simulink model "RobotX_ss_acousticsSKIP_dock_odoa_1021"  (R2014a)
settings: Solver=FixedStepDiscrete  StartTime=0.0  StopTime=inf  FixedStep=.25  RelTol=1e-3
undefined symbols (not defined in the file): Com1, Com2, Com3, Com4, DiscIntNeverNeededParam, standard
libraries: xpcseriallib x42, slrtlib x8, simulink x7, speedgoatlib x2, speedgoatlib_IO102 x1
(part 7 of 19)

== matlab function RobotX_ss_acousticsSKIP_dock_odoa_1021/Main FSM/ODOA/SLAM1/SLAM enabled/slammed ==
  data: mpa output; lm_data input; pre_part_positions input; part_positions output; positionboat input
%% SLAM by Chidananda Matada Shivananda
%  Copyright 2010 Randolph Voorhies

%  Edited 2014 Nick DiLeo - Modifications for unknown data association
%  and multiple measurements in a single timestep
    
%  Edited 2014 Chidananda Matada Shivananda - Simulink compatability, New
%  clustering technique added

%  This program is free software: you can redistribute it and/or modify
%  it under the terms of the GNU General Public License as published by
%  the Free Software Foundation, either version 3 of the License, or
%  (at your option) any later version.
%
%  This program is distributed in the hope that it will be useful,
%  but WITHOUT ANY WARRANTY; without even the implied warranty of
%  MERCHANTABILITY or FITNESS FOR A PARTICULAR PURPOSE.  See the
%  GNU General Public License for more details.
%
%  You should have received a copy of the GNU General Public License
%  along with this program.  If not, see <http://www.gnu.org/licenses/>.

function [mpa,part_positions]   = slammed(lm_data,pre_part_positions,positionboat)

%% General comments

% the angles in radians
% the ditance in m

%% Initialisations.

persistent particles avg_robot;
num_particles = 50;

% the limits
max_read_distance = 10;
min_read_distance = 5;
min_read_angle = -67.5*pi/180; %radians- maximum read angle
max_read_angle = 67.5*pi/180;

% The initial starting position of the robot Use UTM coordinates from GPS
avg_robot_position = [0;0;0];% x y rotation

% The Gaussian variance of the movement commands
% Approximating there are only two drives
% movement_variance = [.1;.1];   % Left drive Right_drive
% M = [movement_variance(1), 0.0;
%      0.0, movement_variance(2)];
measurement_variance = [0.01; 0.01];   % Distance Angle
R = [measurement_variance(1), 0.0;
    0.0, measurement_variance(2)];

default_importance=0.001;

if isempty(particles)
    %  Particles
    %             w[1]
    %             position[1,3]
    %             num_landmarks[300] this is to keep history
    
    %             lm_weight[2,15]based on number of landmarks
    %             landmarks[15]
    %                         position[2,1]
    %                         E[2,2]
    %                         counter[1]
    particles=repmat(struct('w',1.0/num_particles,'position',avg_robot_position,'num_landmarks',zeros(1,2),'lm_weight',repmat(1.0/num_particles,10,15),'landmarks',repmat(struct('pos',zeros(1,2),'E',zeros(2,2),'counter',0),1,15)),1,50);
    avg_robot_position = average_pos(particles,num_particles);
end

if isempty(avg_robot)
    avg_robot=avg_robot_position;
end

avg_robot_position=avg_robot;

%% Upload the moved data onto the particles
for shiva9=1:50
    particles(shiva9).position(1)= pre_part_positions(3*(shiva9-1)+1);
    particles(shiva9).position(2)= pre_part_positions(3*(shiva9-1)+1)*(pi/180);
    particles(shiva9).position(3)= pre_part_positions(3*(shiva9-1)+1);
end

%% Try to take a reading from each landmark and calculate the Jacobian
doResample = false;
% The input got from landmarks
[~,cols]=find(lm_data ~= 0);
if (isempty(cols)==0)% if the cols is not empty
    doResample=true; %if there is new measurement, then resample particles
end

if (doResample==true)
%     [r,~]=size(cols);
    [~,r]=size(cols);
    shiva=1;
    G=zeros(2,2,ceil(r/2));
    z_real=zeros(2,ceil(r/2));
    read_distance=zeros(ceil(r/2));
    read_angle=zeros(ceil(r/2));
    
    for lIdx = 1:2:r %amount of visible landmarks
        real_landmark = [lm_data(cols(lIdx+1)),lm_data(cols(lIdx))];
        % Take a real (noisy) measurement from the robot to the landmark
        %         [z_real(:,lIdx), G(:,:,lIdx)] = getRealMeasurement(avg_robot_position, real_landmark, [0 0]);
        %         function [z, H] = getRealMeasurement(pos, landmark_pos, observation_variance)
        
        landmark_angle=real_landmark(1);
        landmark_distance=real_landmark(2);
        % Compute the Jacobian of this measurement function
        q = landmark_distance^2.0;
        G(:,:,shiva) = [-(real_landmark(1) - avg_robot_position(1))/sqrt(q), -(real_landmark(2) - avg_robot_position(2))/sqrt(q);
            (real_landmark(2) - avg_robot_position(2))/q,       -(real_landmark(1) - avg_robot_position(1))/q];
        
        z_real(:,shiva) = [landmark_distance; landmark_angle];
        read_distance(shiva) = z_real(1,shiva);
        read_angle(shiva)    = z_real(2,shiva);
        shiva=shiva+1;
    end
    %     shiva=1;
    
    for pIdx = 1:num_particles
        %     particles(pIdx).lm_weight=[];
        %     clear z_p H Q
        %         coder.varsize('H', [2,2,16],[0 0 1]);
        num_landmarks=particles(pIdx).num_landmarks(1);
        assert(num_landmarks<20);
        H=zeros(2,2,num_landmarks);
        %         coder.varsize('z_p', [2 1 16]);
        z_p=zeros(2,1,num_landmarks);
        Q=zeros(2,2,num_landmarks);
        for j=1:particles(pIdx).num_landmarks(1)
            %             [z_p(:,j), H(:,:,j)] = getMeasurement(particles(pIdx).position, particles(pIdx).landmarks(j).pos, [0 0]);
            %             function [z, H] = getRealMeasurement(pos, landmark_pos, observation_variance)
            landmark_angle=particles(pIdx).landmarks(j).pos(1);
            landmark_distance=particles(pIdx).landmarks(j).pos(2);
            
            % Compute the Jacobian of this measurement function
            q = landmark_distance^2.0;
            %   H = [-(landmark_pos(1) - pos(1))/sqrt(q), -(landmark_pos(2) - pos(2))/sqrt(q), 0.0;
            %         (landmark_pos(2) - pos(2))/q,       -(landmark_pos(1) - pos(1))/q,      -1.0;
            %         0.0,                                0.0,                               1.0];
            
            H(:,:,j) = [-(particles(pIdx).landmarks(j).pos(1) - particles(pIdx).position(1))/sqrt(q), -(particles(pIdx).landmarks(j).pos(2) - particles(pIdx).position(2))/sqrt(q);
                (particles(pIdx).landmarks(j).pos(2) - particles(pIdx).position(2))/q,       -(particles(pIdx).landmarks(j).pos(1) - particles(pIdx).position(1))/q];
            
            
            z_p(:,j) = [landmark_distance;
                landmark_angle];
            
            for measured_lm=1:size(z_real,2)
                residual = z_real(:,measured_lm) - z_p(:,j);
                Q(:,:,j) = H(:,:,j)' * particles(pIdx).landmarks(j).E * H(:,:,j) + R;
                particles(pIdx).lm_weight(measured_lm,j) = particles(pIdx).w * norm(2*pi*Q(:,:,j)).^(-1/2)*exp(-1/2*(residual'/Q(:,:,j)*residual));
            end
        end
        
        particles(pIdx).num_landmarks(2)=particles(pIdx).num_landmarks(1);
        num_landmarks2=particles(pIdx).num_landmarks(2);
        assert(num_landmarks2<20);
        
        %           clear c_hat
        %         clear cost_table data_associate_mat data_associate_vect
        %%%%%%%%%%%%%%%%%%%%%%%%%%%%%%%%%%%%%%%%%%%%%%%%%%%%%%%%%%%%%%%%%%%%%%%%%%%%%%%%%%%%%%%%%%%%%%%%%%%%%%%%%%%%%%%%%%%%%%%%%%%%%%%%%%%%%%%%%%%%%
        cost_table=zeros(size(z_real,2),num_landmarks+size(z_real,2));
        %         cost_table=zeros(size(z_real,2),num_landmarks);
        
        if (num_landmarks~=0)
            cost_table(1:size(z_real,2),1:particles(pIdx).num_landmarks(1))=particles(pIdx).lm_weight(1:size(z_real,2),1:particles(pIdx).num_landmarks(1));
        end
        cost_table(1:size(z_real,2),particles(pIdx).num_landmarks(1)+1:particles(pIdx).num_landmarks(1)+size(z_real,2)) =default_importance*eye(size(z_real,2));
        
        particles(pIdx).w=max(max(cost_table,[],1),[],2);
        [~, idx_hold]=max(cost_table,[],1); %this is the max correseponding for each measurement
        for i=1:size(cost_table,2)
            idx_zero=setdiff(1:size(cost_table,1),idx_hold(i));
            cost_table(idx_zero,i)=0;
        end
        
        cost_table1=cost_table;
        for shiva14=1:size(cost_table,2)
            cost_table(:,shiva14)=cost_table1(:,size(cost_table,2)-shiva14+1);
        end
        
        
        new_landmarks=0;
        for measured_lm=1:size(z_real,2)
            [~, IDX] = max(cost_table(measured_lm,:));
            if IDX > particles(pIdx).num_landmarks(1)
                new_landmarks=new_landmarks+1;
            end
        end
        
        
        assert(new_landmarks<20);
        data_associate_mat=zeros(size(z_real,2),new_landmarks+num_landmarks2);
        
        for measured_lm=1:size(z_real,2)
            [~, IDX] = max(cost_table(measured_lm,:));
            if IDX > particles(pIdx).num_landmarks(1)
                %we haven't seen this landmark before
                %                 if particles(pIdx).num_landmarks(2)>14
                %                     break;
                %                 end
                particles(pIdx).num_landmarks(2)=particles(pIdx).num_landmarks(2)+1; %add new landmark
                data_associate_mat(measured_lm,particles(pIdx).num_landmarks(2))=measured_lm; %set correspondance b/t measurement and feature j
            else
                %we've already seen this landmark
                %           [val idx]=max(particles(pIdx).lm_weight(measured_lm,:));
                data_associate_mat(measured_lm,IDX)=measured_lm; %measurement is a known feature
            end
            
        end
        
        num_landmarks2=particles(pIdx).num_landmarks(2);
        assert(num_landmarks2<20);
        Hn=zeros(2,2,num_landmarks2);
        t=size(H);
        for i=1:t(3)
            Hn(:,:,i)=H(:,:,i);
        end
        
        %         H=zeros(2,2,num_landmarks2);
        H=Hn;
        
        data_associate_vect=max(data_associate_mat,[],1); %vector that contains measurement correspondance to landmarks
        i=1;
        feature_to_delete=zeros(num_landmarks2);
        for j=1:particles(pIdx).num_landmarks(2) %length(data_associate_vect)
            if (data_associate_vect(j)>0 && j>particles(pIdx).num_landmarks(1))
                % If we have never seen this landmark, then we need to initialize it.
                % We'll just use whatever first reading we recieved.
                particles(pIdx).landmarks(j).pos = [particles(pIdx).position(1) + ...
                    sin(read_angle(data_associate_vect(j))+particles(pIdx).position(3))*read_distance(data_associate_vect(j));...
                    particles(pIdx).position(2) + cos(read_angle(data_associate_vect(j))+particles(pIdx).position(3))*read_distance(data_associate_vect(j))]';
                % Initialize the landmark position covariance
                H(:,:,j)=G(:,:,data_associate_vect(j));
                particles(pIdx).landmarks(j).E = inv(G(:,:,data_associate_vect(j)))' * R * inv(G(:,:,data_associate_vect(j)));
                particles(pIdx).landmarks(j).counter=1; %initialize counter
            elseif (data_associate_vect(j)>0 && j<=particles(pIdx).num_landmarks(1))
                %we've seen this landmark before
                K = particles(pIdx).landmarks(j).E * H(:,:,j) / Q(:,:,j);
                % Mix the ideal reading, and our actual reading using the Kalman gain, and use the result
                % to predict a new landmark position
                particles(pIdx).landmarks(j).pos = particles(pIdx).landmarks(j).pos + (K*(z_real(:,data_associate_vect(j))-z_p(:,j)))';
                % Update the covariance of this landmark
                particles(pIdx).landmarks(j).E = (eye(size(H(:,:,j))) - K*H(:,:,j)')*particles(pIdx).landmarks(j).E;
                particles(pIdx).landmarks(j).counter=particles(pIdx).landmarks(j).counter+1; %increment counter
            else
                % We are leaving these unchanged.  These are commented
                % out, but this is what is actually happening in alg.
                % particles(pIdx).landmarks(j).pos = particles(pIdx).landmarks(j).pos;
                % particles(pIdx).landmarks(j).E=particles(pIdx).landmarks(j).E;
                dist_to_landmark=norm([particles(pIdx).landmarks(j).pos(1)-particles(pIdx).position(1) particles(pIdx).landmarks(j).pos(2)-particles(pIdx).position(2)]);
                ang_to_landmark=atan2((particles(pIdx).landmarks(j).pos(1) - particles(pIdx).position(1)),...
                    (particles(pIdx).landmarks(j).pos(2) - particles(pIdx).position(2)))-particles(pIdx).position(3);
                if (dist_to_landmark > max_read_distance ||dist_to_landmark < min_read_distance || ang_to_landmark > max_read_angle || ang_to_landmark < min_read_angle)
                    %counter(pIdx,j)=counter(pIdx,j) %don't change counter
                else
                    particles(pIdx).landmarks(j).counter=particles(pIdx).landmarks(j).counter-1; %decrement counter
                    if particles(pIdx).landmarks(j).counter<0
                        feature_to_delete(i)=j; %we're going to delete all these features at the end of the loop
                        i=i+1;
                    end
                end
                %
            end %if
        end %end j
        %     'pos',zeros(1,2),'E',zeros(2,2),'counter',0
        if~(isempty(nonzeros(feature_to_delete)))
            tobe_del=nonzeros(feature_to_delete);
            for shiva4=1:length(feature_to_delete)
                particles(pIdx).landmarks(tobe_del(shiva4)).pos=zeros(1,2);
                particles(pIdx).landmarks(tobe_del(shiva4)).E=zeros(2,2);
                particles(pIdx).landmarks(tobe_del(shiva4)).counter=0;
            end
            particles(pIdx).num_landmarks(2)= particles(pIdx).num_landmarks(2)-length(tobe_del);
        end
        
        particles(pIdx).num_landmarks(1)=particles(pIdx).num_landmarks(2);
        
    end %pIdx
    
    particles=resample(particles) ;
    
    
    
end% if (doResample==true)


%% Clustering
landmarks_positions=zeros(15*50,2);
row_counter=0;
for pIdx=1:num_particles
    for j=1:15 %this should be index timestep when in full script
        row_counter=row_counter+1;
        landmarks_positions(row_counter,:)=particles(pIdx).landmarks(j).pos(1:2)';
    end
end

[mpa,]=cluster(landmarks_positions,lm_data,positionboat);
max(landmarks_positions),max(mpa)
% 
% mpadi=mpa(:,1);
% mpaan=((mpa(:,2)));


%% new data prediction

%     lm_data_ind=lm_data(:)~=0;
%     lm_data_ind(1)=0;
%     lm_data1=lm_data(lm_data_ind);
%     
%     for j=(length(lm_data)/2)+1:(length(lm_data))
%         if lm_data(j)<91
%             lm_data(j)=psi(i)+lm_data(j);
%         else
%             lm_data(j)=psi(i)+lm_data(j)-360;
%         end
%     end
%     
%     if length(lm_data~=0)
%         x1=x(i)+(lm_data(1:length(lm_data)/2)/100).*sind(lm_data((length(lm_data)/2)+1:length(lm_data)));
%         y1=y(i)+(lm_data(1:length(lm_data)/2)/100).*cosd(lm_data((length(lm_data)/2)+1:length(lm_data)));
%     end

% landmarks_positions
% mpa1
% mpa=mpa1;




%% Final changes to be persistent
avg_robot=avg_robot_position;
part_positions=zeros(150,1);

for shiva9=1:3:150
    part_positions(shiva9)=particles(ceil(shiva9/3)).position(1);
    part_positions(shiva9+1)=(particles(ceil(shiva9/3)).position(2))*(180/pi);
    part_positions(shiva9+2)=particles(ceil(shiva9/3)).position(3);
end

%% Display and output

end %function [y,y1]  = slammed(imu_data,lm_data)

function [map,mapconv]= cluster(data,lm_add,positionboat)

n=size(data,1);
clusters=ones(n,1);
hubs=zeros(n,1);
hubs(1,1)=1;
dif=zeros(n,2);
% clustersort=zeros(n,3);
for i = 1:n
    dif(i,:)= data(clusters(i),:) - data(i,:);
end

dist =sum((dif.*dif),2);
counter =1;             %Keeps track of number of the present number of hubs
continue12 = 1;   % 1=true 0=false indicates whether to continue forming new
% rearr_lm(:,1)=lm_add(1:2:24)+rand(1);

while continue12
    counter = counter + 1;    % adding new hub
    if counter>750
        break;
    end
    [~,i]=max(dist);        %m= maximum value in the distance array
    %i is the location of the maximum value in the
    % array
    hubs(counter)=i;        %assigns index to new hub
    temp = i*ones(n,1);
    dif1=zeros(n,2);
    for i23 = 1:n
        dif1(i23,:)= data(temp(i23),:) - data(i23,:);
    end
    newdist =sum((dif1.*dif1),2);
    for r=1:n
        if newdist(r) < dist(r)
            dist(r)=newdist(r);
            clusters(r)=i;
        end     %end for if
    end
    maxdist=max(dist);      %returns distance of point farthest from its hub
    continue12 = farout(counter,hubs,data,maxdist); %Checks the stop condition
end

clustersort=[data,clusters];
clustersort=sortrows(clustersort,3);
map=zeros(12,2);
temp=zeros(12,1);
temp(1,1)=clustersort(1,3);
shiva12=1;
for i=1:n
    if sum(temp==clustersort(i,3)) == 0
        shiva12=shiva12+1;
        if shiva12>12
            break
        end
        temp(shiva12)=clustersort(i,3);
    end
end
for shiva13=1:12
    clusterIdx = clustersort(:,3)==temp(shiva13);
    map(shiva13,:)=[sum(clustersort(clusterIdx,1)),sum(clustersort(clusterIdx,2))]/(sum(clusterIdx)*50);
end
map(isnan(map))=0;

x=positionboat(1);
y=positionboat(2);
psi=positionboat(3);
for shiva17=1:2:23
    lm_add(shiva17+1)=lm_add(shiva17+1)*(180/pi);
    if lm_add(shiva17+1)<91
        lm_add(shiva17+1)=psi+lm_add(shiva17+1);
    else
        lm_add(shiva17+1)=psi+lm_add(shiva17+1)-360;
    end
end

shiva18=1;
mapconv=zeros(12,2);
for shiva17=1:2:23
    if (lm_add(shiva17)~=0 && lm_add(shiva17+1)~=0)
        mapconv(shiva18,1)=x+(lm_add(shiva17)*sind(lm_add(shiva17+1)));
        mapconv(shiva18,2)=y+(lm_add(shiva17)*cosd(lm_add(shiva17+1)));
        shiva18=shiva18+1;
    end
end

% map=map.*0.02;
for shiva19=1:12
   if (map(shiva19,1)<1000 && map(shiva19,1)~=0)
       map(shiva19,1)=map(shiva19,1)+4216.58; 
   end
   if (map(shiva19,2)<500 && map(shiva19,1)~=0)
       map(shiva19,2)=map(shiva19,2)+964; 
   end
end
% map(:,1)=map(:,1)+4216.58;
% map(:,2)=map(:,2)+964;
% map=map;
% map=map;
end

function continue1 = farout(counter1,hubs1,data1,maxdist1)

%FAROUT continue = farout(counter,hubs,data,maxdist)
%       Calculates stop condition.  Stops if the point farthest from its
%       hub is within the average distance value.

index1 = 0;
n=size(data1,1);
dif=zeros(n,2);
for i1 = 1:(counter1-1)
    for j = i1+1 : counter1
        index1 = index1 + 1;
        if index1>750
            break
        end
        dif(index1,:)=data1(hubs1(i1),:) - data1(hubs1(j),:);
    end
end

dist=sqrt(sum((dif.*dif),2));
average_dist = sum(dist)/(2*index1);
if (sqrt(maxdist1) < (average_dist/100000))
    continue1 = 0;
else continue1 =1;
end
end                             % end for farout

function avg_robot_position = average_pos(particles,num_particles)
xsiva=0;
ysiva=0;
rotasiva=0;

for siva=1:num_particles
    xsiva=xsiva+particles(siva).position(1);
    ysiva=ysiva+particles(siva).position(2);
    rotasiva=rotasiva+particles(siva).position(3);
end

avg_robot_position = [xsiva/num_particles; ysiva/num_particles; rotasiva/num_particles];

end

function [newParticles] = resample(oldParticles)
% Resample a group of particles such that those with higher weights have a
% higher chance of being replicated, and those with low weights have a high
% chance of disappearing
num_particles=50;
avg_robot_position = [0;0;0];% x y rotation
newParticles=repmat(struct('w',1.0/num_particles,'position',avg_robot_position,'num_landmarks',zeros(1,2),'lm_weight',repmat(1.0/num_particles,10,15),'landmarks',repmat(struct('pos',zeros(1,2),'E',zeros(2,2),'counter',0),1,15)),1,50);

weightSum = 0;
for i=1:length(oldParticles)
    weightSum = weightSum + oldParticles(i).w;
end
for i=1:length(oldParticles)
    oldParticles(i).w = oldParticles(i).w/weightSum;
end
M = length(oldParticles);
%   newParticles = [];
r = rand / M;
c = oldParticles(1).w;
i = 1;
shiva6=1;
assert(shiva6<51);
for m=1:M
    U = r + (m-1) * M^(-1);
    while U > c
        i = i+1;
        c = c+oldParticles(i).w;
    end
    newParticles(shiva6) = oldParticles(i);
    shiva6=shiva6+1;
end
for i=1:length(newParticles)
    newParticles(i).w = 1.0/length(newParticles);
end
end

== system RobotX_ss_acousticsSKIP_dock_odoa_1021/Main FSM/ODOA/Path/Output Reassign ==
  Vaild : Inport
  Data : Inport  Port=2
  Sensors : Inport  Port=3
  Acoustic Active : Constant  Value=0
  Bus Creator2 : BusCreator  Inputs=3
  Bus Creator3 : BusCreator  Inputs=3
  Bus Creator5 : BusCreator  Inputs=2
  Constant3 : Constant  Value=0
  Lidar Mode : Constant  Value=0
  Outputs : Outport
  wires:
  Sensors/1 -> Bus Creator5/2  "Sensors"
  Bus Creator5/1 -> Outputs/1  "Output Signals"
  Vaild/1 -> Bus Creator2/1  "Valid"
  Constant3/1 -> Bus Creator2/2  "Control Mode"
  Data/1 -> Bus Creator2/3  "Data"
  Bus Creator2/1 -> Bus Creator3/1  "Navigation Outputs"
  Acoustic Active/1 -> Bus Creator3/2  "Acoustic Active"
  Lidar Mode/1 -> Bus Creator3/3  "Lidar Mode"
  Bus Creator3/1 -> Bus Creator5/1  "Outputs"

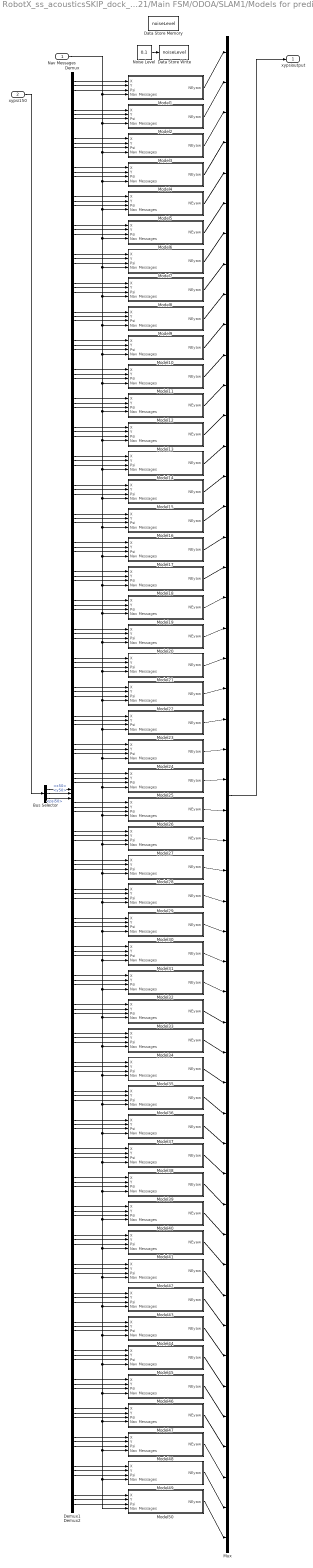
== system RobotX_ss_acousticsSKIP_dock_odoa_1021/Main FSM/ODOA/SLAM1/Models for prediction ==
  Nav Messages : Inport
  xypsi150 : Inport  Port=2
  Bus Selector : BusSelector  OutputSignals=x50,y50,psi50
  Data Store Memory : DataStoreMemory  DataStoreName=noiseLevel  ReadBeforeWriteMsg=warning  WriteAfterWriteMsg=warning  WriteAfterReadMsg=warning
  Data Store Write : DataStoreWrite  DataStoreName=noiseLevel
  Demux : Demux  Outputs=50
  Demux1 : Demux  Outputs=50
  Demux2 : Demux  Outputs=50
  Model1 : Subsystem
  Model10 : Subsystem
  Model11 : Subsystem
  Model12 : Subsystem
  Model13 : Subsystem
  Model14 : Subsystem
  Model15 : Subsystem
  Model16 : Subsystem
  Model17 : Subsystem
  Model18 : Subsystem
  Model19 : Subsystem
  Model2 : Subsystem
  Model20 : Subsystem
  Model21 : Subsystem
  Model22 : Subsystem
  Model23 : Subsystem
  Model24 : Subsystem
  Model25 : Subsystem
  Model26 : Subsystem
  Model27 : Subsystem
  Model28 : Subsystem
  Model29 : Subsystem
  Model3 : Subsystem
  Model30 : Subsystem
  Model31 : Subsystem
  Model32 : Subsystem
  Model33 : Subsystem
  Model34 : Subsystem
  Model35 : Subsystem
  Model36 : Subsystem
  Model37 : Subsystem
  Model38 : Subsystem
  Model39 : Subsystem
  Model4 : Subsystem
  Model40 : Subsystem
  Model41 : Subsystem
  Model42 : Subsystem
  Model43 : Subsystem
  Model44 : Subsystem
  Model45 : Subsystem
  Model46 : Subsystem
  Model47 : Subsystem
  Model48 : Subsystem
  Model49 : Subsystem
  Model5 : Subsystem
  Model50 : Subsystem
  Model6 : Subsystem
  Model7 : Subsystem
  Model8 : Subsystem
  Model9 : Subsystem
  Mux : Mux  Inputs=50
  Noise Level : Constant  Value=0.1
  xypsioutput : Outport  PortDimensions=150
  wires:
  Noise Level/1 -> Data Store Write/1
  Demux/1 -> Model1/1(X)
  Demux1/1 -> Model1/2(Y)
  Demux2/1 -> Model1/3(Psi)
  Demux/2 -> Model2/1(X)
  Demux1/2 -> Model2/2(Y)
  Demux2/2 -> Model2/3(Psi)
  Demux/3 -> Model3/1(X)
  Demux1/3 -> Model3/2(Y)
  Demux2/3 -> Model3/3(Psi)
  Demux/4 -> Model4/1(X)
  Demux1/4 -> Model4/2(Y)
  Demux2/4 -> Model4/3(Psi)
  Demux/5 -> Model5/1(X)
  Demux1/5 -> Model5/2(Y)
  Demux2/5 -> Model5/3(Psi)
  Demux/6 -> Model6/1(X)
  Demux1/6 -> Model6/2(Y)
  Demux2/6 -> Model6/3(Psi)
  Nav Messages/1 -> Model1/4(Nav Messages), Model2/4(Nav Messages), Model3/4(Nav Messages), Model4/4(Nav Messages), Model5/4(Nav Messages), Model6/4(Nav Messages), Model7/4(Nav Messages), Model8/4(Nav Messages), Model9/4(Nav Messages), Model10/4(Nav Messages), Model11/4(Nav Messages), Model12/4(Nav Messages), Model13/4(Nav Messages), Model14/4(Nav Messages), Model15/4(Nav Messages), Model16/4(Nav Messages), Model17/4(Nav Messages), Model18/4(Nav Messages), Model19/4(Nav Messages), Model20/4(Nav Messages), Model21/4(Nav Messages), Model22/4(Nav Messages), Model23/4(Nav Messages), Model24/4(Nav Messages), Model25/4(Nav Messages), Model26/4(Nav Messages), Model27/4(Nav Messages), Model28/4(Nav Messages), Model29/4(Nav Messages), Model30/4(Nav Messages), Model31/4(Nav Messages), Model32/4(Nav Messages), Model33/4(Nav Messages), Model34/4(Nav Messages), Model35/4(Nav Messages), Model36/4(Nav Messages), Model37/4(Nav Messages), Model38/4(Nav Messages), Model39/4(Nav Messages), Model40/4(Nav Messages), Model41/4(Nav Messages), Model42/4(Nav Messages), Model43/4(Nav Messages), Model44/4(Nav Messages), Model45/4(Nav Messages), Model46/4(Nav Messages), Model47/4(Nav Messages), Model48/4(Nav Messages), Model50/4(Nav Messages), Model49/4(Nav Messages)
  Demux2/15 -> Model15/3(Psi)
  Demux1/15 -> Model15/2(Y)
  Demux/15 -> Model15/1(X)
  Demux2/14 -> Model14/3(Psi)
  Demux1/14 -> Model14/2(Y)
  Demux/14 -> Model14/1(X)
  Demux2/13 -> Model13/3(Psi)
  Demux1/13 -> Model13/2(Y)
  Demux/13 -> Model13/1(X)
  Demux2/12 -> Model12/3(Psi)
  Demux1/12 -> Model12/2(Y)
  Demux/12 -> Model12/1(X)
  Demux2/11 -> Model11/3(Psi)
  Demux1/11 -> Model11/2(Y)
  Demux/11 -> Model11/1(X)
  Demux2/10 -> Model10/3(Psi)
  Demux1/10 -> Model10/2(Y)
  Demux/10 -> Model10/1(X)
  Demux2/9 -> Model9/3(Psi)
  Demux1/9 -> Model9/2(Y)
  Demux/9 -> Model9/1(X)
  Demux2/8 -> Model8/3(Psi)
  Demux1/8 -> Model8/2(Y)
  Demux/8 -> Model8/1(X)
  Demux2/7 -> Model7/3(Psi)
  Demux1/7 -> Model7/2(Y)
  Demux/7 -> Model7/1(X)
  Demux/16 -> Model16/1(X)
  Demux1/16 -> Model16/2(Y)
  Demux2/16 -> Model16/3(Psi)
  Demux/17 -> Model17/1(X)
  Demux1/17 -> Model17/2(Y)
  Demux2/17 -> Model17/3(Psi)
  Demux/18 -> Model18/1(X)
  Demux1/18 -> Model18/2(Y)
  Demux2/18 -> Model18/3(Psi)
  Demux/19 -> Model19/1(X)
  Demux1/19 -> Model19/2(Y)
  Demux2/19 -> Model19/3(Psi)
  Demux/20 -> Model20/1(X)
  Demux1/20 -> Model20/2(Y)
  Demux2/20 -> Model20/3(Psi)
  Demux/21 -> Model21/1(X)
  Demux1/21 -> Model21/2(Y)
  Demux2/21 -> Model21/3(Psi)
  Demux/22 -> Model22/1(X)
  Demux1/22 -> Model22/2(Y)
  Demux2/22 -> Model22/3(Psi)
  Demux/23 -> Model23/1(X)
  Demux1/23 -> Model23/2(Y)
  Demux2/23 -> Model23/3(Psi)
  Demux/24 -> Model24/1(X)
  Demux1/24 -> Model24/2(Y)
  Demux2/24 -> Model24/3(Psi)
  Demux/25 -> Model25/1(X)
  Demux1/25 -> Model25/2(Y)
  Demux2/25 -> Model25/3(Psi)
  Demux/26 -> Model26/1(X)
  Demux1/26 -> Model26/2(Y)
  Demux2/26 -> Model26/3(Psi)
  Demux/27 -> Model27/1(X)
  Demux1/27 -> Model27/2(Y)
  Demux2/27 -> Model27/3(Psi)
  Demux/28 -> Model28/1(X)
  Demux1/28 -> Model28/2(Y)
  Demux2/28 -> Model28/3(Psi)
  Demux/29 -> Model29/1(X)
  Demux1/29 -> Model29/2(Y)
  Demux2/29 -> Model29/3(Psi)
  Demux/30 -> Model30/1(X)
  Demux1/30 -> Model30/2(Y)
  Demux2/30 -> Model30/3(Psi)
  Demux/31 -> Model31/1(X)
  Demux1/31 -> Model31/2(Y)
  Demux2/31 -> Model31/3(Psi)
  Demux/32 -> Model32/1(X)
  Demux1/32 -> Model32/2(Y)
  Demux2/32 -> Model32/3(Psi)
  Demux/33 -> Model33/1(X)
  Demux1/33 -> Model33/2(Y)
  Demux2/33 -> Model33/3(Psi)
  Demux/34 -> Model34/1(X)
  Demux1/34 -> Model34/2(Y)
  Demux2/34 -> Model34/3(Psi)
  Demux/35 -> Model35/1(X)
  Demux1/35 -> Model35/2(Y)
  Demux2/35 -> Model35/3(Psi)
  Demux/36 -> Model36/1(X)
  Demux1/36 -> Model36/2(Y)
  Demux2/36 -> Model36/3(Psi)
  Demux/37 -> Model37/1(X)
  Demux1/37 -> Model37/2(Y)
  Demux2/37 -> Model37/3(Psi)
  Demux/38 -> Model38/1(X)
  Demux1/38 -> Model38/2(Y)
  Demux2/38 -> Model38/3(Psi)
  Demux/39 -> Model39/1(X)
  Demux1/39 -> Model39/2(Y)
  Demux2/39 -> Model39/3(Psi)
  Demux/40 -> Model40/1(X)
  Demux1/40 -> Model40/2(Y)
  Demux2/40 -> Model40/3(Psi)
  Demux/41 -> Model41/1(X)
  Demux1/41 -> Model41/2(Y)
  Demux2/41 -> Model41/3(Psi)
  Demux/42 -> Model42/1(X)
  Demux1/42 -> Model42/2(Y)
  Demux2/42 -> Model42/3(Psi)
  Demux/43 -> Model43/1(X)
  Demux1/43 -> Model43/2(Y)
  Demux2/43 -> Model43/3(Psi)
  Demux/44 -> Model44/1(X)
  Demux1/44 -> Model44/2(Y)
  Demux2/44 -> Model44/3(Psi)
  Demux/45 -> Model45/1(X)
  Demux1/45 -> Model45/2(Y)
  Demux2/45 -> Model45/3(Psi)
  Demux/46 -> Model46/1(X)
  Demux1/46 -> Model46/2(Y)
  Demux2/46 -> Model46/3(Psi)
  Demux/47 -> Model47/1(X)
  Demux1/47 -> Model47/2(Y)
  Demux2/47 -> Model47/3(Psi)
  Demux/48 -> Model48/1(X)
  Demux1/48 -> Model48/2(Y)
  Demux2/48 -> Model48/3(Psi)
  Demux/49 -> Model49/1(X)
  Demux1/49 -> Model49/2(Y)
  Demux2/49 -> Model49/3(Psi)
  Demux/50 -> Model50/1(X)
  Demux1/50 -> Model50/2(Y)
  Demux2/50 -> Model50/3(Psi)
  xypsi150/1 -> Bus Selector/1
  Bus Selector/1 -> Demux/1  "<x50>"
  Bus Selector/2 -> Demux1/1  "<y50>"
  Bus Selector/3 -> Demux2/1  "<psi50>"
  Model27/1(NEyaw) -> Mux/27
  Model26/1(NEyaw) -> Mux/26
  Model25/1(NEyaw) -> Mux/25
  Model24/1(NEyaw) -> Mux/24
  Model28/1(NEyaw) -> Mux/28
  Model23/1(NEyaw) -> Mux/23
  Model21/1(NEyaw) -> Mux/21
  Model30/1(NEyaw) -> Mux/30
  Model29/1(NEyaw) -> Mux/29
  Model22/1(NEyaw) -> Mux/22
  Model40/1(NEyaw) -> Mux/40
  Model33/1(NEyaw) -> Mux/33
  Model36/1(NEyaw) -> Mux/36
  Model38/1(NEyaw) -> Mux/38
  Model37/1(NEyaw) -> Mux/37
  Model35/1(NEyaw) -> Mux/35
  Model39/1(NEyaw) -> Mux/39
  Model31/1(NEyaw) -> Mux/31
  Model32/1(NEyaw) -> Mux/32
  Model34/1(NEyaw) -> Mux/34
  Model2/1(NEyaw) -> Mux/2
  Model5/1(NEyaw) -> Mux/5
  Model3/1(NEyaw) -> Mux/3
  Model4/1(NEyaw) -> Mux/4
  Model19/1(NEyaw) -> Mux/19
  Model13/1(NEyaw) -> Mux/13
  Model14/1(NEyaw) -> Mux/14
  Model12/1(NEyaw) -> Mux/12
  Model16/1(NEyaw) -> Mux/16
  Model17/1(NEyaw) -> Mux/17
  Model18/1(NEyaw) -> Mux/18
  Model20/1(NEyaw) -> Mux/20
  Model11/1(NEyaw) -> Mux/11
  Model15/1(NEyaw) -> Mux/15
  Model10/1(NEyaw) -> Mux/10
  Model8/1(NEyaw) -> Mux/8
  Model9/1(NEyaw) -> Mux/9
  Model7/1(NEyaw) -> Mux/7
  Model6/1(NEyaw) -> Mux/6
  Model48/1(NEyaw) -> Mux/48
  Model42/1(NEyaw) -> Mux/42
  Model49/1(NEyaw) -> Mux/49
  Model47/1(NEyaw) -> Mux/47
  Model50/1(NEyaw) -> Mux/50
  Model43/1(NEyaw) -> Mux/43
  Model45/1(NEyaw) -> Mux/45
  Model44/1(NEyaw) -> Mux/44
  Model46/1(NEyaw) -> Mux/46
  Model41/1(NEyaw) -> Mux/41
  Model1/1(NEyaw) -> Mux/1
  Mux/1 -> xypsioutput/1

== system RobotX_ss_acousticsSKIP_dock_odoa_1021/Main FSM/ODOA/SLAM1/SLAM enabled ==
  pre_past_positions : Inport
  lm_data : Inport  Port=2
  positionboat : Inport  Port=3
  Enable : EnablePort
  slammed : MATLAB Function  TreatAsAtomicUnit=on
  mpa : Outport
  part_positions : Outport  Port=2
  wires:
  lm_data/1 -> slammed/1(lm_data)
  pre_past_positions/1 -> slammed/2(pre_part_positions)
  slammed/1(mpa) -> mpa/1
  slammed/2(part_positions) -> part_positions/1
  positionboat/1 -> slammed/3(positionboat)

== system RobotX_ss_acousticsSKIP_dock_odoa_1021/Main FSM/ODOA/SLAM1/inputselection ==
  controlchange : Inport
  xypsi : Inport  Port=2
  Landmarkchange : Inport  Port=3
  part_positions : Inport  Port=4
  xypsi150 : Inport  Port=5
  Bus Creator : BusCreator  Inputs=3
  Delay{,1..4} (5 alike) : Delay  DelayLength=1  InitialCondition=0
  MATLAB Function : MATLAB Function  TreatAsAtomicUnit=on
  last particle positions : Outport
  wires:
  Delay/1 -> MATLAB Function/4(part_positions)
  Delay1/1 -> MATLAB Function/3(xypsi)
  Delay2/1 -> MATLAB Function/5(xypsi150)
  Delay4/1 -> MATLAB Function/1(Landmarkchange)
  Delay3/1 -> MATLAB Function/2(controlchange)
  controlchange/1 -> Delay3/1
  xypsi/1 -> Delay1/1
  part_positions/1 -> Delay/1
  Landmarkchange/1 -> Delay4/1
  xypsi150/1 -> Delay2/1
  MATLAB Function/2(y50) -> Bus Creator/2  "y50"
  MATLAB Function/3(psi50) -> Bus Creator/3  "psi50"
  MATLAB Function/1(x50) -> Bus Creator/1  "x50"
  Bus Creator/1 -> last particle positions/1  "last particle positions"

== system RobotX_ss_acousticsSKIP_dock_odoa_1021/Main FSM/Start//Speedgate/Aim/Output Heirarchy ==
  Data : Inport
  Sensors : Inport  Port=2
  Acoustic Active : Constant  Value=0
  Bus Creator2 : BusCreator  Inputs=3
  Bus Creator3 : BusCreator  Inputs=3
  Bus Creator5 : BusCreator  Inputs=2
  Constant : Constant
  Constant3 : Constant
  Lidar Mode : Constant
  Outputs : Outport
  wires:
  Sensors/1 -> Bus Creator5/2  "Sensors"
  Bus Creator5/1 -> Outputs/1  "Output Signals"
  Constant/1 -> Bus Creator2/1  "Valid"
  Constant3/1 -> Bus Creator2/2  "Control Mode"
  Data/1 -> Bus Creator2/3  "Data"
  Bus Creator2/1 -> Bus Creator3/1  "Navigation Outputs"
  Acoustic Active/1 -> Bus Creator3/2  "Acoustic Active"
  Lidar Mode/1 -> Bus Creator3/3  "Lidar Mode"
  Bus Creator3/1 -> Bus Creator5/1  "Outputs"

== system RobotX_ss_acousticsSKIP_dock_odoa_1021/Main FSM/Start//Speedgate/Dead Reckon/Output Reassign ==
  Vaild : Inport
  Data : Inport  Port=2
  Sensors : Inport  Port=3
  Acoustic Active : Constant  Value=0
  Bus Creator2 : BusCreator  Inputs=3
  Bus Creator3 : BusCreator  Inputs=3
  Bus Creator5 : BusCreator  Inputs=2
  Constant3 : Constant  Value=0
  Lidar Mode : Constant  Value=3
  Outputs : Outport
  wires:
  Sensors/1 -> Bus Creator5/2  "Sensors"
  Bus Creator5/1 -> Outputs/1  "Output Signals"
  Vaild/1 -> Bus Creator2/1  "Valid"
  Constant3/1 -> Bus Creator2/2  "Control Mode"
  Data/1 -> Bus Creator2/3  "Data"
  Bus Creator2/1 -> Bus Creator3/1  "Navigation Outputs"
  Acoustic Active/1 -> Bus Creator3/2  "Acoustic Active"
  Lidar Mode/1 -> Bus Creator3/3  "Lidar Mode"
  Bus Creator3/1 -> Bus Creator5/1  "Outputs"

== system RobotX_ss_acousticsSKIP_dock_odoa_1021/Main FSM/Start//Speedgate/GPS Move/Output Reassign ==
  Vaild : Inport
  Data : Inport  Port=2
  Sensors : Inport  Port=3
  Acoustic Active : Constant  Value=0
  Bus Creator2 : BusCreator  Inputs=3
  Bus Creator3 : BusCreator  Inputs=3
  Bus Creator5 : BusCreator  Inputs=2
  Constant3 : Constant  Value=0
  Lidar Mode : Constant  Value=0
  Outputs : Outport
  wires:
  Sensors/1 -> Bus Creator5/2  "Sensors"
  Bus Creator5/1 -> Outputs/1  "Output Signals"
  Vaild/1 -> Bus Creator2/1  "Valid"
  Constant3/1 -> Bus Creator2/2  "Control Mode"
  Data/1 -> Bus Creator2/3  "Data"
  Bus Creator2/1 -> Bus Creator3/1  "Navigation Outputs"
  Acoustic Active/1 -> Bus Creator3/2  "Acoustic Active"
  Lidar Mode/1 -> Bus Creator3/3  "Lidar Mode"
  Bus Creator3/1 -> Bus Creator5/1  "Outputs"

== system RobotX_ss_acousticsSKIP_dock_odoa_1021/Sensors/1021 Comms/Message Selector/HRT Message ==
  Parameters : Inport
  Time : Inport  Port=2
  Bus Selector : BusSelector  OutputSignals=Sensors.Navigation Message.GPS (LLA).Lat,Sensors.Navigation Message.GPS (LLA).Long,Sensors.Navigation Message.On/Off/RC/Auto,Main Task
  MATLAB Function : MATLAB Function  TreatAsAtomicUnit=on
  HRT Message : Outport
  wires:
  MATLAB Function/1(asciiHRT) -> HRT Message/1
  Parameters/1 -> Bus Selector/1
  Time/1 -> MATLAB Function/1(Time)
  Bus Selector/1 -> MATLAB Function/2(HRTLat)  "<Lat>"
  Bus Selector/2 -> MATLAB Function/3(HRTLong)  "<Long>"
  Bus Selector/3 -> MATLAB Function/4(HRTMode)  "<On/Off/RC/Auto>"
  Bus Selector/4 -> MATLAB Function/5(HRTTask)  "<Main Task>"

== system RobotX_ss_acousticsSKIP_dock_odoa_1021/Sensors/1021 Comms/Message Selector/HRTLIT Message ==
  Parameters : Inport
  Time : Inport  Port=2
  Bus Selector : BusSelector  OutputSignals=Sensors.Navigation Message.GPS (LLA).Lat,Sensors.Navigation Message.GPS (LLA).Long,Main Task,Sensors.Navigation Message.On/Off/RC/Auto
  Data Store Read1 : DataStoreRead  DataStoreName=ltSeq
  MATLAB Function : MATLAB Function  TreatAsAtomicUnit=on
  MATLAB Function1 : MATLAB Function  TreatAsAtomicUnit=on
  HRTLIT Message : Outport
  wires:
  MATLAB Function/1(asciiHRTLIT) -> HRTLIT Message/1
  Time/1 -> MATLAB Function/1(Time)
  Parameters/1 -> Bus Selector/1
  Bus Selector/3 -> MATLAB Function/4(HRTTask)  "<Main Task>"
  Bus Selector/2 -> MATLAB Function/3(HRTLong)  "<Long>"
  Bus Selector/1 -> MATLAB Function/2(HRTLat)  "<Lat>"
  Bus Selector/4 -> MATLAB Function/5(HRTMode)  "<On/Off/RC/Auto>"
  Data Store Read1/1 -> MATLAB Function1/1(ltSeq)
  MATLAB Function1/2(LITSequence) -> MATLAB Function/7(LITSequence)
  MATLAB Function1/1(LITValid) -> MATLAB Function/6(LITValid)

== system RobotX_ss_acousticsSKIP_dock_odoa_1021/Sensors/1021 Comms/Message Selector/HRTSEA Message ==
  Parameters : Inport
  Time : Inport  Port=2
  Bus Selector : BusSelector  OutputSignals=Sensors.Navigation Message.GPS (LLA).Lat,Sensors.Navigation Message.GPS (LLA).Long,Main Task,Sensors.Navigation Message.On/Off/RC/Auto
  Data Store Read3 : DataStoreRead  DataStoreName=pingerInfo
  MATLAB Function : MATLAB Function  TreatAsAtomicUnit=on
  MATLAB Function1 : MATLAB Function  TreatAsAtomicUnit=on
  HRTSEA Message : Outport
  wires:
  MATLAB Function/1(asciiHRTSEA) -> HRTSEA Message/1
  Parameters/1 -> Bus Selector/1
  Time/1 -> MATLAB Function/1(Time)
  Data Store Read3/1 -> MATLAB Function1/1(pingerInfo)
  Bus Selector/3 -> MATLAB Function/4(HRTTask)  "<Main Task>"
  Bus Selector/1 -> MATLAB Function/2(HRTLat)  "<Lat>"
  Bus Selector/2 -> MATLAB Function/3(HRTLong)  "<Long>"
  Bus Selector/4 -> MATLAB Function/5(HRTMode)  "<On/Off/RC/Auto>"
  MATLAB Function1/3(SEALong) -> MATLAB Function/8(SEALong)
  MATLAB Function1/2(SEALat) -> MATLAB Function/7(SEALat)
  MATLAB Function1/5(SEADepth) -> MATLAB Function/10(SEADepth)
  MATLAB Function1/4(SEAColor) -> MATLAB Function/9(SEAColor)
  MATLAB Function1/1(SEAValid) -> MATLAB Function/6(SEAValid)

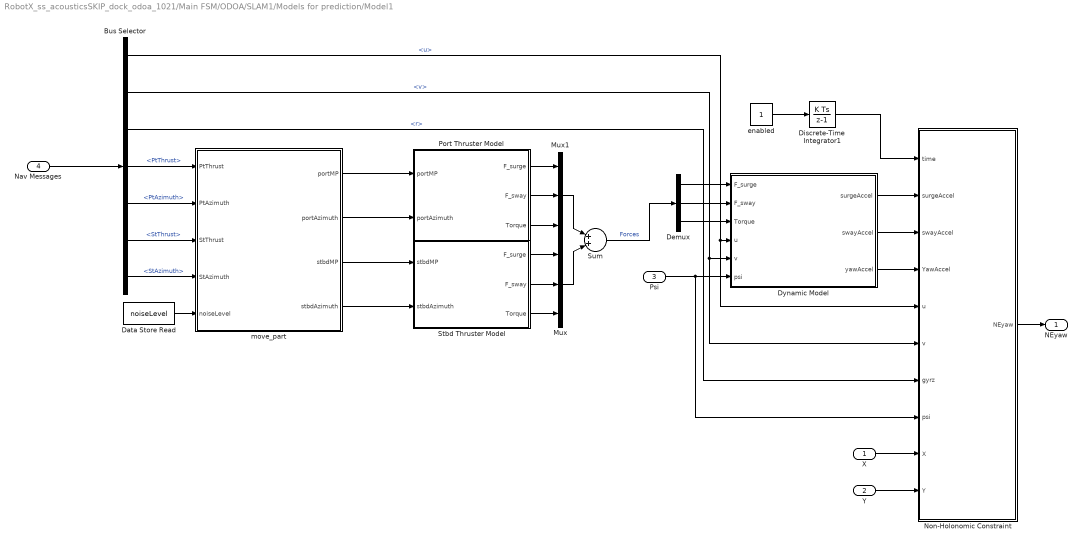
== system RobotX_ss_acousticsSKIP_dock_odoa_1021/Main FSM/ODOA/SLAM1/Models for prediction/Model1 ==
  X : Inport
  Y : Inport  Port=2
  Psi : Inport  Port=3
  Nav Messages : Inport  Port=4
  Bus Selector : BusSelector  OutputSignals=Velocity.u,Velocity.v,Velocity.r,Port.PtThrust,Port.PtAzimuth,Stbd.StThrust,Stbd.StAzimuth
  Data Store Read : DataStoreRead  DataStoreName=noiseLevel
  Demux : Demux  Outputs=3
  Discrete-Time Integrator1 : DiscreteIntegrator  SampleTime=-1  ICPrevOutput=DiscIntNeverNeededParam  ICPrevScaledInput=DiscIntNeverNeededParam
  Dynamic Model : MATLAB Function  TreatAsAtomicUnit=on
  Mux : Mux  Inputs=3
  Mux1 : Mux  Inputs=3
  Non-Holonomic Constraint : MATLAB Function  TreatAsAtomicUnit=on
  Port Thruster Model : MATLAB Function  TreatAsAtomicUnit=on
  Stbd Thruster Model : MATLAB Function  TreatAsAtomicUnit=on
  Sum : Sum  Inputs=|++|
  enabled : Constant
  move_part : MATLAB Function  TreatAsAtomicUnit=on
  NEyaw : Outport
  wires:
  Sum/1 -> Demux/1  "Forces"
  Bus Selector/2 -> Non-Holonomic Constraint/6(v), Dynamic Model/5(v)  "<v>"
  Bus Selector/1 -> Non-Holonomic Constraint/5(u), Dynamic Model/4(u)  "<u>"
  Psi/1 -> Non-Holonomic Constraint/8(psi), Dynamic Model/6(psi)
  Demux/2 -> Dynamic Model/2(F_sway)
  Demux/3 -> Dynamic Model/3(Torque)
  Demux/1 -> Dynamic Model/1(F_surge)
  Mux/1 -> Sum/2
  Stbd Thruster Model/1(F_surge) -> Mux/1
  Stbd Thruster Model/3(Torque) -> Mux/3
  Stbd Thruster Model/2(F_sway) -> Mux/2
  Mux1/1 -> Sum/1
  Port Thruster Model/2(F_sway) -> Mux1/2
  Port Thruster Model/1(F_surge) -> Mux1/1
  Port Thruster Model/3(Torque) -> Mux1/3
  Dynamic Model/1(surgeAccel) -> Non-Holonomic Constraint/2(surgeAccel)
  Dynamic Model/2(swayAccel) -> Non-Holonomic Constraint/3(swayAccel)
  Dynamic Model/3(yawAccel) -> Non-Holonomic Constraint/4(YawAccel)
  Y/1 -> Non-Holonomic Constraint/10(Y)
  X/1 -> Non-Holonomic Constraint/9(X)
  Bus Selector/3 -> Non-Holonomic Constraint/7(gyrz)  "<r>"
  Non-Holonomic Constraint/1(NEyaw) -> NEyaw/1
  enabled/1 -> Discrete-Time Integrator1/1
  Discrete-Time Integrator1/1 -> Non-Holonomic Constraint/1(time)
  Nav Messages/1 -> Bus Selector/1
  Bus Selector/4 -> move_part/1(PtThrust)  "<PtThrust>"
  Bus Selector/5 -> move_part/2(PtAzimuth)  "<PtAzimuth>"
  Bus Selector/7 -> move_part/4(StAzimuth)  "<StAzimuth>"
  Bus Selector/6 -> move_part/3(StThrust)  "<StThrust>"
  move_part/1(portMP) -> Port Thruster Model/1(portMP)
  move_part/2(portAzimuth) -> Port Thruster Model/2(portAzimuth)
  move_part/3(stbdMP) -> Stbd Thruster Model/1(stbdMP)
  move_part/4(stbdAzimuth) -> Stbd Thruster Model/2(stbdAzimuth)
  Data Store Read/1 -> move_part/5(noiseLevel)

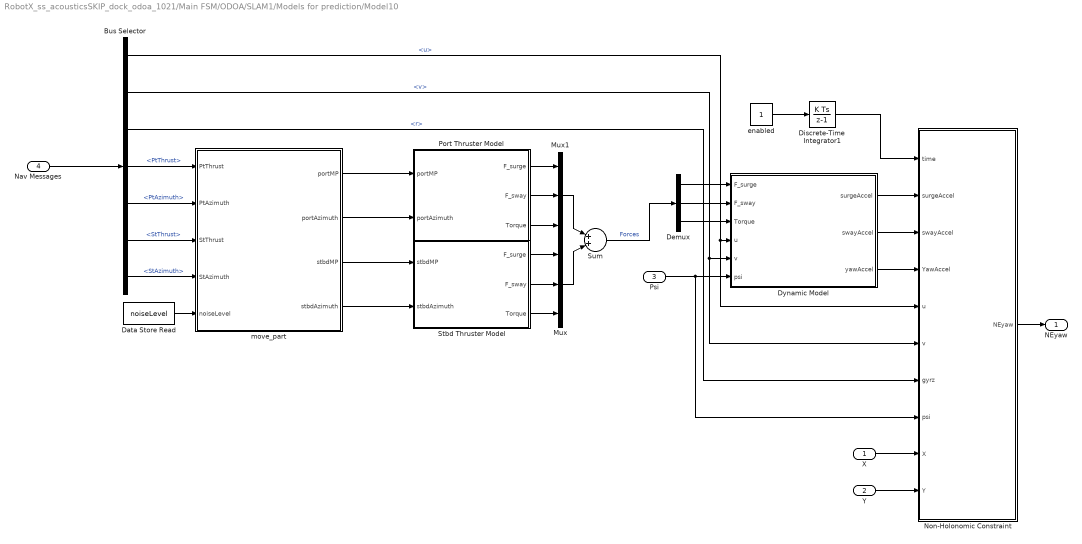
== system RobotX_ss_acousticsSKIP_dock_odoa_1021/Main FSM/ODOA/SLAM1/Models for prediction/Model10 ==
  X : Inport
  Y : Inport  Port=2
  Psi : Inport  Port=3
  Nav Messages : Inport  Port=4
  Bus Selector : BusSelector  OutputSignals=Velocity.u,Velocity.v,Velocity.r,Port.PtThrust,Port.PtAzimuth,Stbd.StThrust,Stbd.StAzimuth
  Data Store Read : DataStoreRead  DataStoreName=noiseLevel
  Demux : Demux  Outputs=3
  Discrete-Time Integrator1 : DiscreteIntegrator  SampleTime=-1  ICPrevOutput=DiscIntNeverNeededParam  ICPrevScaledInput=DiscIntNeverNeededParam
  Dynamic Model : MATLAB Function  TreatAsAtomicUnit=on
  Mux : Mux  Inputs=3
  Mux1 : Mux  Inputs=3
  Non-Holonomic Constraint : MATLAB Function  TreatAsAtomicUnit=on
  Port Thruster Model : MATLAB Function  TreatAsAtomicUnit=on
  Stbd Thruster Model : MATLAB Function  TreatAsAtomicUnit=on
  Sum : Sum  Inputs=|++|
  enabled : Constant
  move_part : MATLAB Function  TreatAsAtomicUnit=on
  NEyaw : Outport
  wires:
  Sum/1 -> Demux/1  "Forces"
  Bus Selector/2 -> Non-Holonomic Constraint/6(v), Dynamic Model/5(v)  "<v>"
  Bus Selector/1 -> Non-Holonomic Constraint/5(u), Dynamic Model/4(u)  "<u>"
  Psi/1 -> Non-Holonomic Constraint/8(psi), Dynamic Model/6(psi)
  Demux/2 -> Dynamic Model/2(F_sway)
  Demux/3 -> Dynamic Model/3(Torque)
  Demux/1 -> Dynamic Model/1(F_surge)
  Mux/1 -> Sum/2
  Stbd Thruster Model/1(F_surge) -> Mux/1
  Stbd Thruster Model/3(Torque) -> Mux/3
  Stbd Thruster Model/2(F_sway) -> Mux/2
  Mux1/1 -> Sum/1
  Port Thruster Model/2(F_sway) -> Mux1/2
  Port Thruster Model/1(F_surge) -> Mux1/1
  Port Thruster Model/3(Torque) -> Mux1/3
  Dynamic Model/1(surgeAccel) -> Non-Holonomic Constraint/2(surgeAccel)
  Dynamic Model/2(swayAccel) -> Non-Holonomic Constraint/3(swayAccel)
  Dynamic Model/3(yawAccel) -> Non-Holonomic Constraint/4(YawAccel)
  Y/1 -> Non-Holonomic Constraint/10(Y)
  X/1 -> Non-Holonomic Constraint/9(X)
  Bus Selector/3 -> Non-Holonomic Constraint/7(gyrz)  "<r>"
  Non-Holonomic Constraint/1(NEyaw) -> NEyaw/1
  enabled/1 -> Discrete-Time Integrator1/1
  Discrete-Time Integrator1/1 -> Non-Holonomic Constraint/1(time)
  Nav Messages/1 -> Bus Selector/1
  Bus Selector/4 -> move_part/1(PtThrust)  "<PtThrust>"
  Bus Selector/5 -> move_part/2(PtAzimuth)  "<PtAzimuth>"
  Bus Selector/7 -> move_part/4(StAzimuth)  "<StAzimuth>"
  Bus Selector/6 -> move_part/3(StThrust)  "<StThrust>"
  move_part/1(portMP) -> Port Thruster Model/1(portMP)
  move_part/2(portAzimuth) -> Port Thruster Model/2(portAzimuth)
  move_part/3(stbdMP) -> Stbd Thruster Model/1(stbdMP)
  move_part/4(stbdAzimuth) -> Stbd Thruster Model/2(stbdAzimuth)
  Data Store Read/1 -> move_part/5(noiseLevel)

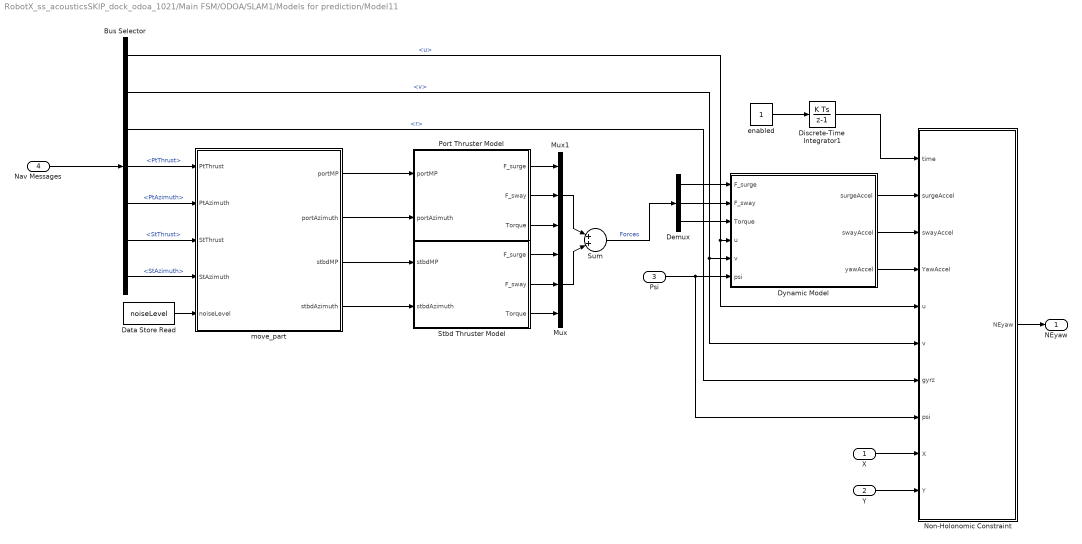
== system RobotX_ss_acousticsSKIP_dock_odoa_1021/Main FSM/ODOA/SLAM1/Models for prediction/Model11 ==
  X : Inport
  Y : Inport  Port=2
  Psi : Inport  Port=3
  Nav Messages : Inport  Port=4
  Bus Selector : BusSelector  OutputSignals=Velocity.u,Velocity.v,Velocity.r,Port.PtThrust,Port.PtAzimuth,Stbd.StThrust,Stbd.StAzimuth
  Data Store Read : DataStoreRead  DataStoreName=noiseLevel
  Demux : Demux  Outputs=3
  Discrete-Time Integrator1 : DiscreteIntegrator  SampleTime=-1  ICPrevOutput=DiscIntNeverNeededParam  ICPrevScaledInput=DiscIntNeverNeededParam
  Dynamic Model : MATLAB Function  TreatAsAtomicUnit=on
  Mux : Mux  Inputs=3
  Mux1 : Mux  Inputs=3
  Non-Holonomic Constraint : MATLAB Function  TreatAsAtomicUnit=on
  Port Thruster Model : MATLAB Function  TreatAsAtomicUnit=on
  Stbd Thruster Model : MATLAB Function  TreatAsAtomicUnit=on
  Sum : Sum  Inputs=|++|
  enabled : Constant
  move_part : MATLAB Function  TreatAsAtomicUnit=on
  NEyaw : Outport
  wires:
  Sum/1 -> Demux/1  "Forces"
  Bus Selector/2 -> Non-Holonomic Constraint/6(v), Dynamic Model/5(v)  "<v>"
  Bus Selector/1 -> Non-Holonomic Constraint/5(u), Dynamic Model/4(u)  "<u>"
  Psi/1 -> Non-Holonomic Constraint/8(psi), Dynamic Model/6(psi)
  Demux/2 -> Dynamic Model/2(F_sway)
  Demux/3 -> Dynamic Model/3(Torque)
  Demux/1 -> Dynamic Model/1(F_surge)
  Mux/1 -> Sum/2
  Stbd Thruster Model/1(F_surge) -> Mux/1
  Stbd Thruster Model/3(Torque) -> Mux/3
  Stbd Thruster Model/2(F_sway) -> Mux/2
  Mux1/1 -> Sum/1
  Port Thruster Model/2(F_sway) -> Mux1/2
  Port Thruster Model/1(F_surge) -> Mux1/1
  Port Thruster Model/3(Torque) -> Mux1/3
  Dynamic Model/1(surgeAccel) -> Non-Holonomic Constraint/2(surgeAccel)
  Dynamic Model/2(swayAccel) -> Non-Holonomic Constraint/3(swayAccel)
  Dynamic Model/3(yawAccel) -> Non-Holonomic Constraint/4(YawAccel)
  Y/1 -> Non-Holonomic Constraint/10(Y)
  X/1 -> Non-Holonomic Constraint/9(X)
  Bus Selector/3 -> Non-Holonomic Constraint/7(gyrz)  "<r>"
  Non-Holonomic Constraint/1(NEyaw) -> NEyaw/1
  enabled/1 -> Discrete-Time Integrator1/1
  Discrete-Time Integrator1/1 -> Non-Holonomic Constraint/1(time)
  Nav Messages/1 -> Bus Selector/1
  Bus Selector/4 -> move_part/1(PtThrust)  "<PtThrust>"
  Bus Selector/5 -> move_part/2(PtAzimuth)  "<PtAzimuth>"
  Bus Selector/7 -> move_part/4(StAzimuth)  "<StAzimuth>"
  Bus Selector/6 -> move_part/3(StThrust)  "<StThrust>"
  move_part/1(portMP) -> Port Thruster Model/1(portMP)
  move_part/2(portAzimuth) -> Port Thruster Model/2(portAzimuth)
  move_part/3(stbdMP) -> Stbd Thruster Model/1(stbdMP)
  move_part/4(stbdAzimuth) -> Stbd Thruster Model/2(stbdAzimuth)
  Data Store Read/1 -> move_part/5(noiseLevel)

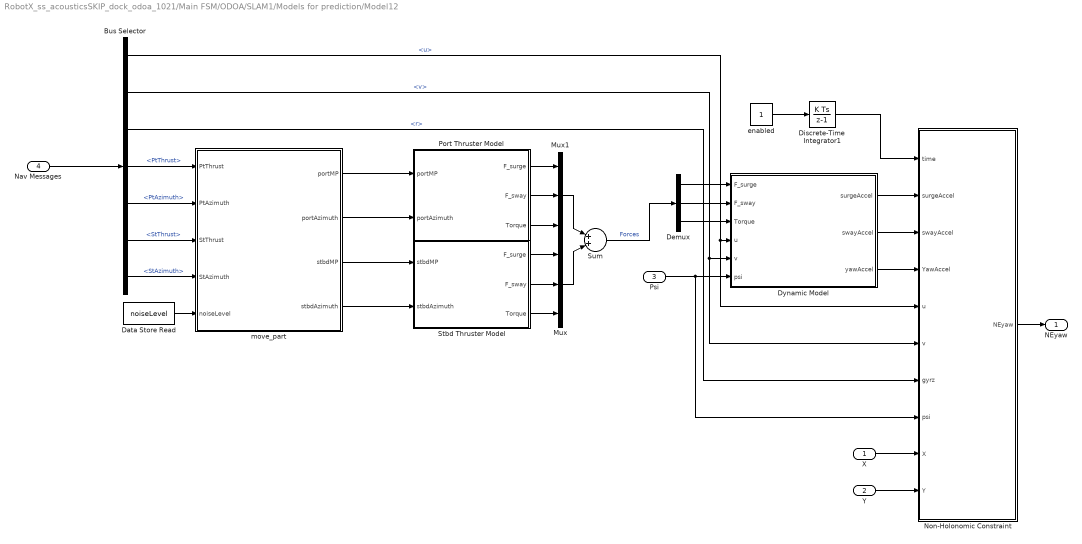
== system RobotX_ss_acousticsSKIP_dock_odoa_1021/Main FSM/ODOA/SLAM1/Models for prediction/Model12 ==
  X : Inport
  Y : Inport  Port=2
  Psi : Inport  Port=3
  Nav Messages : Inport  Port=4
  Bus Selector : BusSelector  OutputSignals=Velocity.u,Velocity.v,Velocity.r,Port.PtThrust,Port.PtAzimuth,Stbd.StThrust,Stbd.StAzimuth
  Data Store Read : DataStoreRead  DataStoreName=noiseLevel
  Demux : Demux  Outputs=3
  Discrete-Time Integrator1 : DiscreteIntegrator  SampleTime=-1  ICPrevOutput=DiscIntNeverNeededParam  ICPrevScaledInput=DiscIntNeverNeededParam
  Dynamic Model : MATLAB Function  TreatAsAtomicUnit=on
  Mux : Mux  Inputs=3
  Mux1 : Mux  Inputs=3
  Non-Holonomic Constraint : MATLAB Function  TreatAsAtomicUnit=on
  Port Thruster Model : MATLAB Function  TreatAsAtomicUnit=on
  Stbd Thruster Model : MATLAB Function  TreatAsAtomicUnit=on
  Sum : Sum  Inputs=|++|
  enabled : Constant
  move_part : MATLAB Function  TreatAsAtomicUnit=on
  NEyaw : Outport
  wires:
  Sum/1 -> Demux/1  "Forces"
  Bus Selector/2 -> Non-Holonomic Constraint/6(v), Dynamic Model/5(v)  "<v>"
  Bus Selector/1 -> Non-Holonomic Constraint/5(u), Dynamic Model/4(u)  "<u>"
  Psi/1 -> Non-Holonomic Constraint/8(psi), Dynamic Model/6(psi)
  Demux/2 -> Dynamic Model/2(F_sway)
  Demux/3 -> Dynamic Model/3(Torque)
  Demux/1 -> Dynamic Model/1(F_surge)
  Mux/1 -> Sum/2
  Stbd Thruster Model/1(F_surge) -> Mux/1
  Stbd Thruster Model/3(Torque) -> Mux/3
  Stbd Thruster Model/2(F_sway) -> Mux/2
  Mux1/1 -> Sum/1
  Port Thruster Model/2(F_sway) -> Mux1/2
  Port Thruster Model/1(F_surge) -> Mux1/1
  Port Thruster Model/3(Torque) -> Mux1/3
  Dynamic Model/1(surgeAccel) -> Non-Holonomic Constraint/2(surgeAccel)
  Dynamic Model/2(swayAccel) -> Non-Holonomic Constraint/3(swayAccel)
  Dynamic Model/3(yawAccel) -> Non-Holonomic Constraint/4(YawAccel)
  Y/1 -> Non-Holonomic Constraint/10(Y)
  X/1 -> Non-Holonomic Constraint/9(X)
  Bus Selector/3 -> Non-Holonomic Constraint/7(gyrz)  "<r>"
  Non-Holonomic Constraint/1(NEyaw) -> NEyaw/1
  enabled/1 -> Discrete-Time Integrator1/1
  Discrete-Time Integrator1/1 -> Non-Holonomic Constraint/1(time)
  Nav Messages/1 -> Bus Selector/1
  Bus Selector/4 -> move_part/1(PtThrust)  "<PtThrust>"
  Bus Selector/5 -> move_part/2(PtAzimuth)  "<PtAzimuth>"
  Bus Selector/7 -> move_part/4(StAzimuth)  "<StAzimuth>"
  Bus Selector/6 -> move_part/3(StThrust)  "<StThrust>"
  move_part/1(portMP) -> Port Thruster Model/1(portMP)
  move_part/2(portAzimuth) -> Port Thruster Model/2(portAzimuth)
  move_part/3(stbdMP) -> Stbd Thruster Model/1(stbdMP)
  move_part/4(stbdAzimuth) -> Stbd Thruster Model/2(stbdAzimuth)
  Data Store Read/1 -> move_part/5(noiseLevel)
